simulink model "twomass"  (R2023b)
settings: Solver=FixedStepAuto  StartTime=0.0  StopTime=10  FixedStep=.05  RelTol=1e-3
settings Model: Creator=dherrin  LastModifiedBy=Todd McKenzie
settings OptimizationCC: ReuseModelBlockBuffer=off

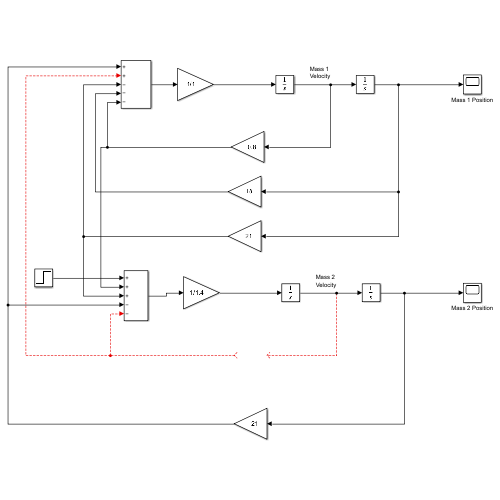
[thumbnail: Simulink's stored preview of the top-level diagram]
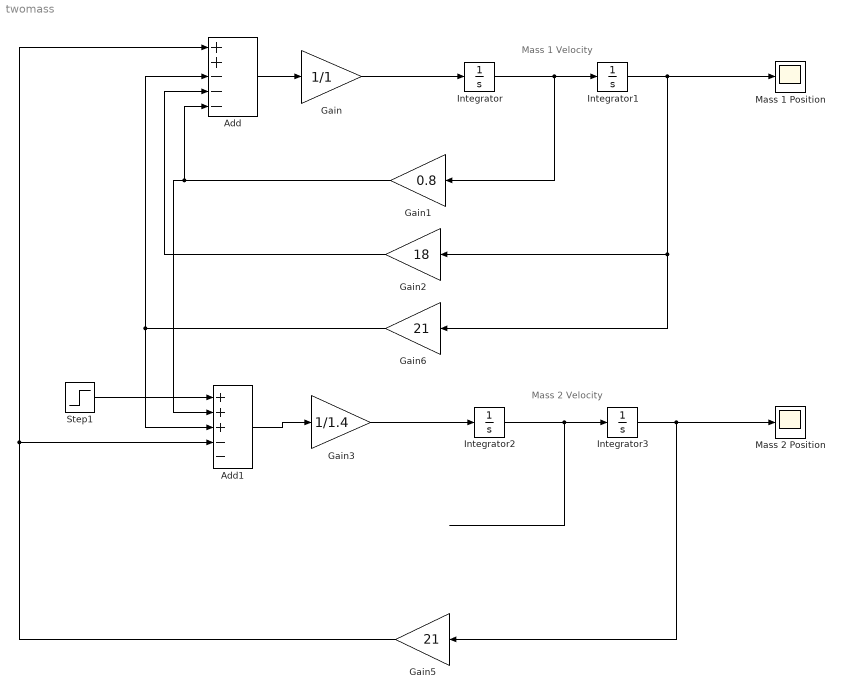
== system twomass ==
  note: Mass 1
      | Velocity
  note: Mass 2
      | Velocity
  Add : Sum  Inputs=++---
  Add1 : Sum  Inputs=+++--
  Gain : Gain  Gain=1/1
  Gain1 : Gain  Gain=0.8
  Gain2 : Gain  Gain=18
  Gain3 : Gain  Gain=1/1.4
  Gain5 : Gain  Gain=21
  Gain6 : Gain  Gain=21
  Integrator : Integrator
  Integrator1 : Integrator  InitialCondition=0.1
  Integrator2 : Integrator
  Integrator3 : Integrator  InitialCondition=-0.1
  Mass 1 Position : Scope
  Mass 2 Position : Scope
  Step1 : Step  Time=0  After=0  SampleTime=0
  wires:
  Gain/1 -> Integrator/1
  Integrator/1 -> Gain1/1, Integrator1/1
  Integrator1/1 -> Gain6/1, Gain2/1, Mass 1 Position/1
  Add/1 -> Gain/1
  Gain2/1 -> Add/4
  ? -> Add1/5, Add/2
  Add1/1 -> Gain3/1
  Integrator2/1 -> Integrator3/1
  Gain5/1 -> Add/1, Add1/4
  Step1/1 -> Add1/1
  Integrator3/1 -> Gain5/1, Mass 2 Position/1
  Gain3/1 -> Integrator2/1
  Gain6/1 -> Add1/3, Add/3
  Gain1/1 -> Add1/2, Add/5
